simulink model "softMBD"  (R2025b)
settings: Solver=FixedStepAuto  StartTime=0.0  StopTime=10  FixedStep=0.005  RelTol=1e-3
values from neighbouring files (symbols this model uses):
  FPV_mass = 0.5    [Soft.m]
  g = 9.81    [Soft.m]
  ks = 0    [Soft.m]
  p_0 = 1013.25    [Soft.m]
  Q2Ts = forcetomotors()    [Soft.m]    (also in forcetomotors.m = inv(Ts2Q))
  takeOffDuration = 2    [Soft.m]
  Ts = 0.005    [Soft.m]
undefined symbols (not defined in the file or in its folder): DiscIntNeverNeededParam, pInitialization, sigbuilder_block
libraries: simulink x34, discretizing x11, slpidlib x2, shared6dof x1, dynamicsLibrary x1, aerolibasang x1, aerolibnav x1
(part 20 of 20)

== system softMBD/FCS/Controller/position_controller/PID Controller3/Anti-windup/Disc. Clamping Ideal/Dead Zone/External ==
  preSat : Inport
  Upper Limit : Inport  Port=2  SampleTime=SampleTime
  Lower Limit : Inport  Port=3  SampleTime=SampleTime
  Dead Zone Dynamic : simulink/Discontinuities/Dead Zone Dynamic
  DZ out : Outport
  wires:
  Dead Zone Dynamic/1 -> DZ out/1
  Upper Limit/1 -> Dead Zone Dynamic/1
  Lower Limit/1 -> Dead Zone Dynamic/3
  preSat/1 -> Dead Zone Dynamic/2

== system softMBD/FCS/Controller/position_controller/PID Controller3/Anti-windup/Disc. Clamping Parallel/Dead Zone/Disabled ==

== system softMBD/FCS/Controller/position_controller/PID Controller3/Anti-windup/Disc. Clamping Parallel/Dead Zone/Enabled ==
  preSat : Inport
  DeadZone : DeadZone  DisableCoverage=on  LowerValue=LowerSaturationLimit  UpperValue=UpperSaturationLimit  SaturateOnIntegerOverflow=off
  DZ out : Outport
  wires:
  DeadZone/1 -> DZ out/1
  preSat/1 -> DeadZone/1

== system softMBD/FCS/Controller/position_controller/PID Controller3/Anti-windup/Disc. Clamping Parallel/Dead Zone/External ==
  preSat : Inport
  Upper Limit : Inport  Port=2  SampleTime=SampleTime
  Lower Limit : Inport  Port=3  SampleTime=SampleTime
  Dead Zone Dynamic : simulink/Discontinuities/Dead Zone Dynamic
  DZ out : Outport
  wires:
  Dead Zone Dynamic/1 -> DZ out/1
  Upper Limit/1 -> Dead Zone Dynamic/1
  Lower Limit/1 -> Dead Zone Dynamic/3
  preSat/1 -> Dead Zone Dynamic/2

== system softMBD/FCS/Controller/position_controller/PID Controller3/Filter/Differentiator/Tsamp/External Ts ==
  U : Inport  SampleTime=SampleTime
  Ts : Inport  Port=2  SampleTime=SampleTime
  Udiff*Ts Prod Out : Product  Inputs=*/  OutMin=UdiffTsProdOutMin  OutMax=UdiffTsProdOutMax  SampleTime=SampleTime
  Out1 : Outport  SampleTime=SampleTime
  wires:
  U/1 -> Udiff*Ts Prod Out/1
  Udiff*Ts Prod Out/1 -> Out1/1
  Ts/1 -> Udiff*Ts Prod Out/2

== system softMBD/FCS/Controller/position_controller/PID Controller3/Filter/Differentiator/Tsamp/Internal Ts ==
  U : Inport  SampleTime=SampleTime
  Ts : Inport  Port=2  SampleTime=SampleTime
  Terminator : Terminator
  Tsamp : SampleTimeMath  TsampMathOp=/  TsampMathImp=Offline Scaling Adjustment
  Out1 : Outport  SampleTime=SampleTime
  wires:
  U/1 -> Tsamp/1
  Ts/1 -> Terminator/1
  Tsamp/1 -> Out1/1

== system softMBD/FCS/Controller/position_controller/PID Controller3/Filter/Disc. Backward Euler Filter/Tsamp/External Ts ==
  N : Inport  SampleTime=SampleTime
  Ts : Inport  Port=2  SampleTime=SampleTime
  N*Ts Prod Out : Product  OutMin=NTsProdOutMin  OutMax=NTsProdOutMax  SampleTime=SampleTime
  Out1 : Outport  SampleTime=SampleTime
  wires:
  Ts/1 -> N*Ts Prod Out/2
  N*Ts Prod Out/1 -> Out1/1
  N/1 -> N*Ts Prod Out/1

== system softMBD/FCS/Controller/position_controller/PID Controller3/Filter/Disc. Backward Euler Filter/Tsamp/Internal Ts ==
  N : Inport  SampleTime=SampleTime
  Ts : Inport  Port=2  SampleTime=SampleTime
  Terminator : Terminator
  Tsamp : SampleTimeMath  TsampMathOp=*
  Out1 : Outport  SampleTime=SampleTime
  wires:
  Tsamp/1 -> Out1/1
  Ts/1 -> Terminator/1
  N/1 -> Tsamp/1

== system softMBD/FCS/Controller/position_controller/PID Controller3/Filter/Disc. Backward Euler Filter Only/Tsamp/External Ts ==
  N : Inport  SampleTime=SampleTime
  Ts : Inport  Port=2  SampleTime=SampleTime
  N*Ts Prod Out : Product  OutMin=NTsProdOutMin  OutMax=NTsProdOutMax  SampleTime=SampleTime
  Out1 : Outport  SampleTime=SampleTime
  wires:
  N/1 -> N*Ts Prod Out/1
  N*Ts Prod Out/1 -> Out1/1
  Ts/1 -> N*Ts Prod Out/2

== system softMBD/FCS/Controller/position_controller/PID Controller3/Filter/Disc. Backward Euler Filter Only/Tsamp/Internal Ts ==
  N : Inport  SampleTime=SampleTime
  Ts : Inport  Port=2  SampleTime=SampleTime
  Terminator : Terminator
  Tsamp : SampleTimeMath  TsampMathOp=*
  Out1 : Outport  SampleTime=SampleTime
  wires:
  N/1 -> Tsamp/1
  Ts/1 -> Terminator/1
  Tsamp/1 -> Out1/1

== system softMBD/FCS/Controller/position_controller/PID Controller3/Filter/Disc. Trapezoidal Filter/Tsamp/External Ts ==
  N : Inport  SampleTime=SampleTime
  Ts : Inport  Port=2  SampleTime=SampleTime
  Gain : Gain  Gain=0.5
  N*Ts Prod Out : Product  OutMin=NTsProdOutMin  OutMax=NTsProdOutMax  SampleTime=SampleTime
  Out1 : Outport  SampleTime=SampleTime
  wires:
  Gain/1 -> N*Ts Prod Out/2
  Ts/1 -> Gain/1
  N*Ts Prod Out/1 -> Out1/1
  N/1 -> N*Ts Prod Out/1

== system softMBD/FCS/Controller/position_controller/PID Controller3/Filter/Disc. Trapezoidal Filter/Tsamp/Internal Ts ==
  N : Inport  SampleTime=SampleTime
  Ts : Inport  Port=2  SampleTime=SampleTime
  Terminator : Terminator
  Tsamp : SampleTimeMath  TsampMathOp=*  weightValue=0.5
  Out1 : Outport  SampleTime=SampleTime
  wires:
  Tsamp/1 -> Out1/1
  Ts/1 -> Terminator/1
  N/1 -> Tsamp/1

== system softMBD/FCS/Controller/position_controller/PID Controller3/Filter/Disc. Trapezoidal Filter Only/Tsamp/External Ts ==
  N : Inport  SampleTime=SampleTime
  Ts : Inport  Port=2  SampleTime=SampleTime
  Gain : Gain  Gain=0.5
  N*Ts Prod Out : Product  OutMin=NTsProdOutMin  OutMax=NTsProdOutMax  SampleTime=SampleTime
  Out1 : Outport  SampleTime=SampleTime
  wires:
  N/1 -> N*Ts Prod Out/1
  N*Ts Prod Out/1 -> Out1/1
  Ts/1 -> Gain/1
  Gain/1 -> N*Ts Prod Out/2

== system softMBD/FCS/Controller/position_controller/PID Controller3/Filter/Disc. Trapezoidal Filter Only/Tsamp/Internal Ts ==
  N : Inport  SampleTime=SampleTime
  Ts : Inport  Port=2  SampleTime=SampleTime
  Terminator : Terminator
  Tsamp : SampleTimeMath  TsampMathOp=*  weightValue=0.5
  Out1 : Outport  SampleTime=SampleTime
  wires:
  N/1 -> Tsamp/1
  Ts/1 -> Terminator/1
  Tsamp/1 -> Out1/1

== system softMBD/FCS/Controller/roll_pitch_controller/PID Controller/Anti-windup/Cont. Clamping Ideal/Dead Zone/Disabled ==

== system softMBD/FCS/Controller/roll_pitch_controller/PID Controller/Anti-windup/Cont. Clamping Ideal/Dead Zone/Enabled ==
  preSat : Inport
  DeadZone : DeadZone  DisableCoverage=on  LowerValue=LowerSaturationLimit  UpperValue=UpperSaturationLimit  SaturateOnIntegerOverflow=off
  DZ out : Outport
  wires:
  preSat/1 -> DeadZone/1
  DeadZone/1 -> DZ out/1

== system softMBD/FCS/Controller/roll_pitch_controller/PID Controller/Anti-windup/Cont. Clamping Ideal/Dead Zone/External ==
  preSat : Inport
  Upper Limit : Inport  Port=2  SampleTime=SampleTime
  Lower Limit : Inport  Port=3  SampleTime=SampleTime
  Dead Zone Dynamic : simulink/Discontinuities/Dead Zone Dynamic
  DZ out : Outport
  wires:
  preSat/1 -> Dead Zone Dynamic/2
  Lower Limit/1 -> Dead Zone Dynamic/3
  Upper Limit/1 -> Dead Zone Dynamic/1
  Dead Zone Dynamic/1 -> DZ out/1

== system softMBD/FCS/Controller/roll_pitch_controller/PID Controller/Anti-windup/Cont. Clamping Parallel/Dead Zone/Disabled ==

== system softMBD/FCS/Controller/roll_pitch_controller/PID Controller/Anti-windup/Cont. Clamping Parallel/Dead Zone/Enabled ==
  preSat : Inport
  DeadZone : DeadZone  DisableCoverage=on  LowerValue=LowerSaturationLimit  UpperValue=UpperSaturationLimit  SaturateOnIntegerOverflow=off
  DZ out : Outport
  wires:
  preSat/1 -> DeadZone/1
  DeadZone/1 -> DZ out/1

== system softMBD/FCS/Controller/roll_pitch_controller/PID Controller/Anti-windup/Cont. Clamping Parallel/Dead Zone/External ==
  preSat : Inport
  Upper Limit : Inport  Port=2  SampleTime=SampleTime
  Lower Limit : Inport  Port=3  SampleTime=SampleTime
  Dead Zone Dynamic : simulink/Discontinuities/Dead Zone Dynamic
  DZ out : Outport
  wires:
  preSat/1 -> Dead Zone Dynamic/2
  Lower Limit/1 -> Dead Zone Dynamic/3
  Upper Limit/1 -> Dead Zone Dynamic/1
  Dead Zone Dynamic/1 -> DZ out/1

== system softMBD/FCS/Controller/roll_pitch_controller/PID Controller/Anti-windup/Disc. Clamping Ideal/Dead Zone/Disabled ==

== system softMBD/FCS/Controller/roll_pitch_controller/PID Controller/Anti-windup/Disc. Clamping Ideal/Dead Zone/Enabled ==
  preSat : Inport
  DeadZone : DeadZone  DisableCoverage=on  LowerValue=LowerSaturationLimit  UpperValue=UpperSaturationLimit  SaturateOnIntegerOverflow=off
  DZ out : Outport
  wires:
  DeadZone/1 -> DZ out/1
  preSat/1 -> DeadZone/1

== system softMBD/FCS/Controller/roll_pitch_controller/PID Controller/Anti-windup/Disc. Clamping Ideal/Dead Zone/External ==
  preSat : Inport
  Upper Limit : Inport  Port=2  SampleTime=SampleTime
  Lower Limit : Inport  Port=3  SampleTime=SampleTime
  Dead Zone Dynamic : simulink/Discontinuities/Dead Zone Dynamic
  DZ out : Outport
  wires:
  Dead Zone Dynamic/1 -> DZ out/1
  Upper Limit/1 -> Dead Zone Dynamic/1
  Lower Limit/1 -> Dead Zone Dynamic/3
  preSat/1 -> Dead Zone Dynamic/2

== system softMBD/FCS/Controller/roll_pitch_controller/PID Controller/Anti-windup/Disc. Clamping Parallel/Dead Zone/Disabled ==

== system softMBD/FCS/Controller/roll_pitch_controller/PID Controller/Anti-windup/Disc. Clamping Parallel/Dead Zone/Enabled ==
  preSat : Inport
  DeadZone : DeadZone  DisableCoverage=on  LowerValue=LowerSaturationLimit  UpperValue=UpperSaturationLimit  SaturateOnIntegerOverflow=off
  DZ out : Outport
  wires:
  DeadZone/1 -> DZ out/1
  preSat/1 -> DeadZone/1

== system softMBD/FCS/Controller/roll_pitch_controller/PID Controller/Anti-windup/Disc. Clamping Parallel/Dead Zone/External ==
  preSat : Inport
  Upper Limit : Inport  Port=2  SampleTime=SampleTime
  Lower Limit : Inport  Port=3  SampleTime=SampleTime
  Dead Zone Dynamic : simulink/Discontinuities/Dead Zone Dynamic
  DZ out : Outport
  wires:
  Dead Zone Dynamic/1 -> DZ out/1
  Upper Limit/1 -> Dead Zone Dynamic/1
  Lower Limit/1 -> Dead Zone Dynamic/3
  preSat/1 -> Dead Zone Dynamic/2

== system softMBD/FCS/Controller/roll_pitch_controller/PID Controller/Filter/Differentiator/Tsamp/External Ts ==
  U : Inport  SampleTime=SampleTime
  Ts : Inport  Port=2  SampleTime=SampleTime
  Udiff*Ts Prod Out : Product  Inputs=*/  OutMin=UdiffTsProdOutMin  OutMax=UdiffTsProdOutMax  SampleTime=SampleTime
  Out1 : Outport  SampleTime=SampleTime
  wires:
  U/1 -> Udiff*Ts Prod Out/1
  Udiff*Ts Prod Out/1 -> Out1/1
  Ts/1 -> Udiff*Ts Prod Out/2

== system softMBD/FCS/Controller/roll_pitch_controller/PID Controller/Filter/Differentiator/Tsamp/Internal Ts ==
  U : Inport  SampleTime=SampleTime
  Ts : Inport  Port=2  SampleTime=SampleTime
  Terminator : Terminator
  Tsamp : SampleTimeMath  TsampMathOp=/  TsampMathImp=Offline Scaling Adjustment
  Out1 : Outport  SampleTime=SampleTime
  wires:
  U/1 -> Tsamp/1
  Ts/1 -> Terminator/1
  Tsamp/1 -> Out1/1

== system softMBD/FCS/Controller/roll_pitch_controller/PID Controller/Filter/Disc. Backward Euler Filter/Tsamp/External Ts ==
  N : Inport  SampleTime=SampleTime
  Ts : Inport  Port=2  SampleTime=SampleTime
  N*Ts Prod Out : Product  OutMin=NTsProdOutMin  OutMax=NTsProdOutMax  SampleTime=SampleTime
  Out1 : Outport  SampleTime=SampleTime
  wires:
  Ts/1 -> N*Ts Prod Out/2
  N*Ts Prod Out/1 -> Out1/1
  N/1 -> N*Ts Prod Out/1

== system softMBD/FCS/Controller/roll_pitch_controller/PID Controller/Filter/Disc. Backward Euler Filter/Tsamp/Internal Ts ==
  N : Inport  SampleTime=SampleTime
  Ts : Inport  Port=2  SampleTime=SampleTime
  Terminator : Terminator
  Tsamp : SampleTimeMath  TsampMathOp=*
  Out1 : Outport  SampleTime=SampleTime
  wires:
  Tsamp/1 -> Out1/1
  Ts/1 -> Terminator/1
  N/1 -> Tsamp/1

== system softMBD/FCS/Controller/roll_pitch_controller/PID Controller/Filter/Disc. Backward Euler Filter Only/Tsamp/External Ts ==
  N : Inport  SampleTime=SampleTime
  Ts : Inport  Port=2  SampleTime=SampleTime
  N*Ts Prod Out : Product  OutMin=NTsProdOutMin  OutMax=NTsProdOutMax  SampleTime=SampleTime
  Out1 : Outport  SampleTime=SampleTime
  wires:
  N/1 -> N*Ts Prod Out/1
  N*Ts Prod Out/1 -> Out1/1
  Ts/1 -> N*Ts Prod Out/2

== system softMBD/FCS/Controller/roll_pitch_controller/PID Controller/Filter/Disc. Backward Euler Filter Only/Tsamp/Internal Ts ==
  N : Inport  SampleTime=SampleTime
  Ts : Inport  Port=2  SampleTime=SampleTime
  Terminator : Terminator
  Tsamp : SampleTimeMath  TsampMathOp=*
  Out1 : Outport  SampleTime=SampleTime
  wires:
  N/1 -> Tsamp/1
  Ts/1 -> Terminator/1
  Tsamp/1 -> Out1/1

== system softMBD/FCS/Controller/roll_pitch_controller/PID Controller/Filter/Disc. Trapezoidal Filter/Tsamp/External Ts ==
  N : Inport  SampleTime=SampleTime
  Ts : Inport  Port=2  SampleTime=SampleTime
  Gain : Gain  Gain=0.5
  N*Ts Prod Out : Product  OutMin=NTsProdOutMin  OutMax=NTsProdOutMax  SampleTime=SampleTime
  Out1 : Outport  SampleTime=SampleTime
  wires:
  Gain/1 -> N*Ts Prod Out/2
  Ts/1 -> Gain/1
  N*Ts Prod Out/1 -> Out1/1
  N/1 -> N*Ts Prod Out/1

== system softMBD/FCS/Controller/roll_pitch_controller/PID Controller/Filter/Disc. Trapezoidal Filter/Tsamp/Internal Ts ==
  N : Inport  SampleTime=SampleTime
  Ts : Inport  Port=2  SampleTime=SampleTime
  Terminator : Terminator
  Tsamp : SampleTimeMath  TsampMathOp=*  weightValue=0.5
  Out1 : Outport  SampleTime=SampleTime
  wires:
  Tsamp/1 -> Out1/1
  Ts/1 -> Terminator/1
  N/1 -> Tsamp/1

== system softMBD/FCS/Controller/roll_pitch_controller/PID Controller/Filter/Disc. Trapezoidal Filter Only/Tsamp/External Ts ==
  N : Inport  SampleTime=SampleTime
  Ts : Inport  Port=2  SampleTime=SampleTime
  Gain : Gain  Gain=0.5
  N*Ts Prod Out : Product  OutMin=NTsProdOutMin  OutMax=NTsProdOutMax  SampleTime=SampleTime
  Out1 : Outport  SampleTime=SampleTime
  wires:
  N/1 -> N*Ts Prod Out/1
  N*Ts Prod Out/1 -> Out1/1
  Ts/1 -> Gain/1
  Gain/1 -> N*Ts Prod Out/2

== system softMBD/FCS/Controller/roll_pitch_controller/PID Controller/Filter/Disc. Trapezoidal Filter Only/Tsamp/Internal Ts ==
  N : Inport  SampleTime=SampleTime
  Ts : Inport  Port=2  SampleTime=SampleTime
  Terminator : Terminator
  Tsamp : SampleTimeMath  TsampMathOp=*  weightValue=0.5
  Out1 : Outport  SampleTime=SampleTime
  wires:
  N/1 -> Tsamp/1
  Ts/1 -> Terminator/1
  Tsamp/1 -> Out1/1

== system softMBD/FCS/filters/Subsystem/x,y,z,dy,dy,dz/z,dz/Kalman Filter1/CalculatePL/DataTypeConversionL ==
  DTS reference : Inport
  u : Inport  Port=2
  Conversion : DataTypeConversion  SaturateOnIntegerOverflow=off  RndMeth=Floor  LockScale=on
  Data Type Duplicate : DataTypeDuplicate  DisableCoverage=on
  y : Outport
  wires:
  Conversion/1 -> Data Type Duplicate/2, y/1
  DTS reference/1 -> Data Type Duplicate/1
  u/1 -> Conversion/1

== system softMBD/FCS/filters/Subsystem/x,y,z,dy,dy,dz/z,dz/Kalman Filter1/CalculatePL/DataTypeConversionM ==
  DTS reference : Inport
  u : Inport  Port=2
  Conversion : DataTypeConversion  SaturateOnIntegerOverflow=off  RndMeth=Floor  LockScale=on
  Data Type Duplicate : DataTypeDuplicate  DisableCoverage=on
  y : Outport
  wires:
  Conversion/1 -> Data Type Duplicate/2, y/1
  DTS reference/1 -> Data Type Duplicate/1
  u/1 -> Conversion/1

== system softMBD/FCS/filters/Subsystem/x,y,z,dy,dy,dz/z,dz/Kalman Filter1/CalculatePL/DataTypeConversionP ==
  DTS reference : Inport
  u : Inport  Port=2
  Conversion : DataTypeConversion  SaturateOnIntegerOverflow=off  RndMeth=Floor  LockScale=on
  Data Type Duplicate : DataTypeDuplicate  DisableCoverage=on
  y : Outport
  wires:
  Conversion/1 -> Data Type Duplicate/2, y/1
  DTS reference/1 -> Data Type Duplicate/1
  u/1 -> Conversion/1

== system softMBD/FCS/filters/Subsystem/x,y,z,dy,dy,dz/z,dz/Kalman Filter1/CalculatePL/DataTypeConversionZ ==
  DTS reference : Inport
  u : Inport  Port=2
  Conversion : DataTypeConversion  SaturateOnIntegerOverflow=off  RndMeth=Floor  LockScale=on
  Data Type Duplicate : DataTypeDuplicate  DisableCoverage=on
  y : Outport
  wires:
  Conversion/1 -> Data Type Duplicate/2, y/1
  DTS reference/1 -> Data Type Duplicate/1
  u/1 -> Conversion/1

== system softMBD/FCS/filters/Subsystem/x,y,z,dy,dy,dz/z,dz/Kalman Filter1/CalculatePL/Ground ==
  note: Specification is to avoid underspecified data type warnings in the code generation process
  Ground : Ground
  Signal Specification : SignalSpecification  OutDataTypeStr=single  Dimensions=1
  Out : Outport  VectorParamsAs1DForOutWhenUnconnected=off
  wires:
  Signal Specification/1 -> Out/1
  Ground/1 -> Signal Specification/1

== system softMBD/FCS/filters/Subsystem/x,y,z,dy,dy,dz/z,dz/Kalman Filter1/CalculateYhat/Ground ==
  note: Specification is to avoid underspecified data type warnings in the code generation process
  Ground : Ground
  Signal Specification : SignalSpecification  OutDataTypeStr=single  Dimensions=1
  Out : Outport  VectorParamsAs1DForOutWhenUnconnected=off
  wires:
  Signal Specification/1 -> Out/1
  Ground/1 -> Signal Specification/1

== system softMBD/FCS/filters/Subsystem/x,y,z,dy,dy,dz/z,dz/Kalman Filter1/CovarianceOutputConfigurator/decideOutput ==
  Z : Inport
  SqrtUsedFcn : MATLAB Function  TreatAsAtomicUnit=on
  isSqrtUsed : Constant  Value=pInitialization.isSqrtUsed  VectorParams1D=off  OutDataTypeStr=boolean
  P : Outport
  wires:
  SqrtUsedFcn/1(P) -> P/1
  Z/1 -> SqrtUsedFcn/1(u)
  isSqrtUsed/1 -> SqrtUsedFcn/2(isSqrtUsed)

== system softMBD/FCS/filters/Subsystem/x,y,z,dy,dy,dz/z,dz/Kalman Filter1/Observer/MeasurementUpdate ==
  L[k] : Inport
  y[k] : Inport  Port=2
  C[k] : Inport  Port=3
  xhat[k|k-1] : Inport  Port=4
  D[k] : Inport  Port=5
  u[k] : Inport  Port=6
  Enable : EnablePort
  Add1 : Sum
  C[k]*xhat[k|k-1] : Product  Multiplication=Matrix(*)
  D[k]*u[k] : Product  Multiplication=Matrix(*)
  Product3 : Product  Multiplication=Matrix(*)
  Sum : Sum  Inputs=|+-
  L*(y[k]-yhat[k|k-1]) : Outport  OutputWhenDisabled=reset  InitialOutput=0  VectorParamsAs1DForOutWhenUnconnected=off
  wires:
  u[k]/1 -> D[k]*u[k]/2
  D[k]/1 -> D[k]*u[k]/1
  xhat[k|k-1]/1 -> C[k]*xhat[k|k-1]/2
  C[k]/1 -> C[k]*xhat[k|k-1]/1
  C[k]*xhat[k|k-1]/1 -> Add1/1
  D[k]*u[k]/1 -> Add1/2
  Add1/1 -> Sum/2  "yhat[k|k-1]"
  Sum/1 -> Product3/2
  y[k]/1 -> Sum/1
  Product3/1 -> L*(y[k]-yhat[k|k-1])/1
  L[k]/1 -> Product3/1

== system softMBD/FCS/filters/Subsystem/x,y,z,dy,dy,dz/z,dz/Kalman Filter1/ReducedQRN/Ground ==
  note: Specification is to avoid underspecified data type warnings in the code generation process
  Ground : Ground
  Signal Specification : SignalSpecification  OutDataTypeStr=single  Dimensions=1
  Out : Outport  VectorParamsAs1DForOutWhenUnconnected=off
  wires:
  Signal Specification/1 -> Out/1
  Ground/1 -> Signal Specification/1

== system softMBD/FCS/filters/Subsystem/x,y,z,dy,dy,dz/z,dz/Kalman Filter1/UseCurrentEstimator/Enabled Subsystem ==
  M[k] : Inport
  C[k] : Inport  Port=2
  y[k] : Inport  Port=3
  xhat[k|k-1] : Inport  Port=4
  Enable : EnablePort
  Add1 : Sum  Inputs=+-
  Product : Product  Multiplication=Matrix(*)
  Product2 : Product  Multiplication=Matrix(*)
  deltax : Outport  OutputWhenDisabled=reset  InitialOutput=0  VectorParamsAs1DForOutWhenUnconnected=off
  wires:
  Product2/1 -> deltax/1
  M[k]/1 -> Product2/1
  Add1/1 -> Product2/2
  y[k]/1 -> Add1/1
  xhat[k|k-1]/1 -> Product/2
  C[k]/1 -> Product/1
  Product/1 -> Add1/2

== matlab function softMBD/FCS/Controller/position_controller/Position error transformation (Earth to Body frame) ==
  data: yaw input; xy_err_earth input; xy_err_body output
function xy_err_body = fcn(yaw,xy_err_earth)

transformation = [cos(yaw), sin(yaw); -sin(yaw),  cos(yaw)];
xy_err_body = transformation * xy_err_earth;


end

== matlab function softMBD/FCS/filters/Subsystem1/roll_kalman/Kalman Filter/CovarianceOutputConfigurator/decideOutput/SqrtUsedFcn ==
  data: u input; P output; isSqrtUsed input
function P = outputCovariance(u,isSqrtUsed)
   
   % Determine if the Square-Root algorithm was used
   if isSqrtUsed
      P = u*u.';
   else
      P = u;
   end   
end

== matlab function softMBD/FCS/filters/Subsystem/x,y,z,dy,dy,dz/z,dz/Kalman Filter1/CovarianceOutputConfigurator/decideOutput/SqrtUsedFcn ==
  data: u input; P output; isSqrtUsed input
function P = outputCovariance(u,isSqrtUsed)
   
   % Determine if the Square-Root algorithm was used
   if isSqrtUsed
      P = u*u.';
   else
      P = u;
   end   
end

== matlab function softMBD/FCS/filters/Subsystem1/pitch_kalman/Kalman Filter1/CovarianceOutputConfigurator/decideOutput/SqrtUsedFcn ==
  data: u input; P output; isSqrtUsed input
function P = outputCovariance(u,isSqrtUsed)
   
   % Determine if the Square-Root algorithm was used
   if isSqrtUsed
      P = u*u.';
   else
      P = u;
   end   
end
